simulink model "m2018"  (R2016a)
settings: Solver=VariableStepAuto  StartTime=0.0  StopTime=0.05  RelTol=1e-3
settings Model: Creator=witkey721  LastModifiedBy=witkey721

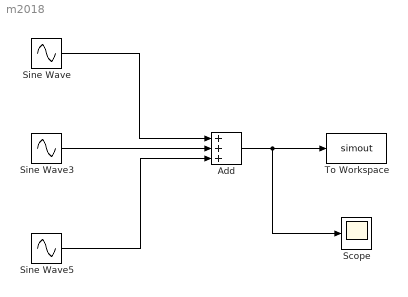
== system m2018 ==
  Add : Sum  Inputs=+++
  Scope : Scope
  Sine Wave : Sin  Frequency=2*pi*50  SampleTime=0
  Sine Wave3 : Sin  Amplitude=1/10  Frequency=3*50*2*pi  SampleTime=0
  Sine Wave5 : Sin  Amplitude=1/100  Frequency=5*50*2*pi  SampleTime=0
  To Workspace : ToWorkspace  VariableName=simout  SaveFormat=Timeseries  SampleTime=-1
  wires:
  Add/1 -> Scope/1, To Workspace/1
  Sine Wave/1 -> Add/1
  Sine Wave3/1 -> Add/2
  Sine Wave5/1 -> Add/3
